simulink model "quindici"  (R2023a)
settings: Solver=VariableStepAuto  StartTime=0.0  StopTime=10*((2*pi)/w)  MaxStep=((2*pi)/w)/1000  RelTol=1e-3
model workspace (MAT data in the model file):
  R1 = 30
  R2 = 15
  R3 = 4
  R4 = 6
  XC = -16
  XL1 = 18
  XL2 = 18
  XM = 9
  a = 2
  w = 6.28318530718
libraries: fl_lib x16, nesl_utility x5
settings Model: Creator=Aguer  LastModifiedBy=Aguer

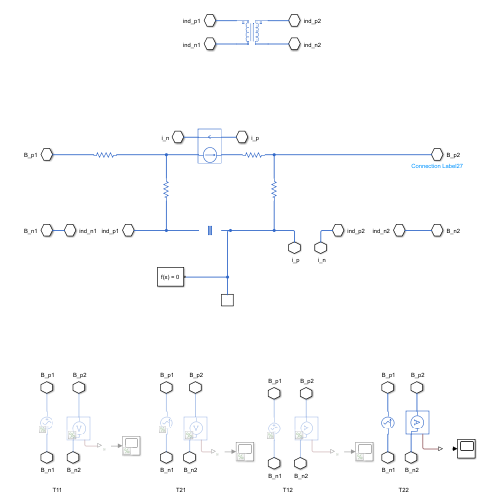
[thumbnail: Simulink's stored preview of the top-level diagram]
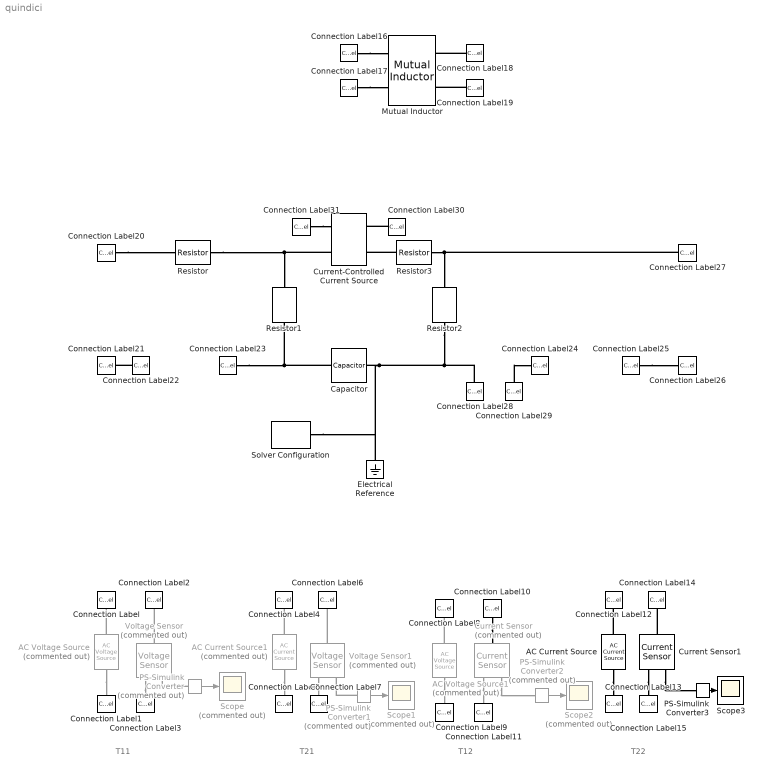
== system quindici ==
  note: T21
  note: T11
  note: T12
  note: T22
  AC Current Source : fl_lib/Electrical/Electrical Sources/AC Current Source  amp=1 A  shift=90 deg  frequency=w/(2*pi) Hz  omega=0 rad/s
      settings: InternalSimscapePortConfiguration="{\"Bottom\":[],\"Left\":[{\"id\":\"p\",\"label\":\"\",\"type\":\"foundation.electrical.electrical\"}],\"Right\":[{\"id\":\"n\",\"label\":\"\",\"type\":\"foundation.electrical.electrical\"}],\"Top\":[]}"
  AC Current Source1 : fl_lib/Electrical/Electrical Sources/AC Current Source  Commented=on  amp=1 A  shift=90 deg  frequency=w/(2*pi) Hz  omega=0 rad/s
      settings: InternalSimscapePortConfiguration="{\"Bottom\":[],\"Left\":[{\"id\":\"p\",\"label\":\"\",\"type\":\"foundation.electrical.electrical\"}],\"Right\":[{\"id\":\"n\",\"label\":\"\",\"type\":\"foundation.electrical.electrical\"}],\"Top\":[]}"
  AC Voltage Source : fl_lib/Electrical/Electrical Sources/AC Voltage Source  Commented=on  amp=1 V  shift=90 deg  frequency=w/(2*pi) Hz  omega=0 rad/s
  AC Voltage Source1 : fl_lib/Electrical/Electrical Sources/AC Voltage Source  Commented=on  amp=1 V  shift=90 deg  frequency=w/(2*pi) Hz  omega=0 rad/s
  Capacitor : fl_lib/Electrical/Electrical Elements/Capacitor  c=-1/(w*XC) F  r=0 Ohm  g=0 1/Ohm  i_specify=off  i_priority=None  i=0 A  i_nominal_specify=off  i_nominal_unit=A  i_nominal_value=1  v_specify=off  v_priority=None  v=0 V  v_nominal_specify=off  v_nominal_unit=V  v_nominal_value=1  vc_specify=off  vc_priority=High  vc=0 V  vc_nominal_specify=off  vc_nominal_unit=V  vc_nominal_value=1
  Connection Label{,4,8,12,20} (5 alike) : ConnectionLabel  Label=B_p1
  Connection Label{1,5,9,13,21} (5 alike) : ConnectionLabel  Label=B_n1
  Connection Label{2,6,10,14,27} (5 alike) : ConnectionLabel  Label=B_p2
  Connection Label{3,7,11,15,26} (5 alike) : ConnectionLabel  Label=B_n2
  Connection Label16 : ConnectionLabel  Label=ind_p1
  Connection Label17 : ConnectionLabel  Label=ind_n1
  Connection Label18 : ConnectionLabel  Label=ind_p2
  Connection Label19 : ConnectionLabel  Label=ind_n2
  Connection Label22 : ConnectionLabel  Label=ind_n1
  Connection Label23 : ConnectionLabel  Label=ind_p1
  Connection Label24 : ConnectionLabel  Label=ind_p2
  Connection Label25 : ConnectionLabel  Label=ind_n2
  Connection Label28 : ConnectionLabel  Label=i_p
  Connection Label29 : ConnectionLabel  Label=i_n
  Connection Label30 : ConnectionLabel  Label=i_p
  Connection Label31 : ConnectionLabel  Label=i_n
  Current Sensor : fl_lib/Electrical/Electrical Sensors/Current Sensor  Commented=on
  Current Sensor1 : fl_lib/Electrical/Electrical Sensors/Current Sensor
  Current-Controlled Current Source : fl_lib/Electrical/Electrical Sources/Current-Controlled Current Source  K=a  i1_specify=off  i1_priority=None  i1=0 A  i1_nominal_specify=off  i1_nominal_unit=A  i1_nominal_value=1  i2_specify=off  i2_priority=None  i2=0 A  i2_nominal_specify=off  i2_nominal_unit=A  i2_nominal_value=1
      settings: InternalSimscapePortConfiguration="{\"Bottom\":[],\"Left\":[{\"id\":\"p1\",\"label\":\"+\",\"type\":\"foundation.electrical.electrical\"},{\"id\":\"head\",\"label\":\"\",\"type\":\"foundation.electrical.electrical\"}],\"Right\":[{\"id\":\"n1\",\"label\":\"-\",\"type\":\"foundation.electrical.electrical\"},{\"id\":\"tail\",\"label\":\"\",\"type\":\"foundation.electrical.electrical\"}],\"Top\":[]}"
  Electrical Reference : fl_lib/Electrical/Electrical Elements/Electrical Reference
  Mutual Inductor : fl_lib/Electrical/Electrical Elements/Mutual Inductor  L1=XL1/w H  L2=XL2/w H  k=XM/XL1  i1_specify=off  i1_priority=High  i1=0 A  i1_nominal_specify=off  i1_nominal_unit=A  i1_nominal_value=1  i2_specify=off  i2_priority=High  i2=0 A  i2_nominal_specify=off  i2_nominal_unit=A  i2_nominal_value=1  v1_specify=off  v1_priority=None  v1=0 V  v1_nominal_specify=off  v1_nominal_unit=V  v1_nominal_value=1  v2_specify=off  v2_priority=None  v2=0 V  v2_nominal_specify=off  v2_nominal_unit=V  v2_nominal_value=1
      settings: InternalSimscapePortConfiguration="{\"Bottom\":[],\"Left\":[{\"id\":\"p1\",\"label\":\"1+\",\"type\":\"foundation.electrical.electrical\"},{\"id\":\"n1\",\"label\":\"1-\",\"type\":\"foundation.electrical.electrical\"}],\"Right\":[{\"id\":\"p2\",\"label\":\"2+\",\"type\":\"foundation.electrical.electrical\"},{\"id\":\"n2\",\"label\":\"2-\",\"type\":\"foundation.electrical.electrical\"}],\"Top\":[]}"
  PS-Simulink Converter : nesl_utility/PS-Simulink Converter  Commented=on  PhysicalDomain=network_engine_domain  SubClassName=ps_output  LeftPortType=input  RightPortType=output  PseudoPeriodic=off  Frequencies=[]  VectorFormat=inherit  Unit=inherit  AffineConversion=off
  PS-Simulink Converter1 : nesl_utility/PS-Simulink Converter  Commented=on  PhysicalDomain=network_engine_domain  SubClassName=ps_output  LeftPortType=input  RightPortType=output  PseudoPeriodic=off  Frequencies=[]  VectorFormat=inherit  Unit=inherit  AffineConversion=off
  PS-Simulink Converter2 : nesl_utility/PS-Simulink Converter  Commented=on  PhysicalDomain=network_engine_domain  SubClassName=ps_output  LeftPortType=input  RightPortType=output  PseudoPeriodic=off  Frequencies=[]  VectorFormat=inherit  Unit=inherit  AffineConversion=off
  PS-Simulink Converter3 : nesl_utility/PS-Simulink Converter  PhysicalDomain=network_engine_domain  SubClassName=ps_output  LeftPortType=input  RightPortType=output  PseudoPeriodic=off  Frequencies=[]  VectorFormat=inherit  Unit=inherit  AffineConversion=off
  Resistor : fl_lib/Electrical/Electrical Elements/Resistor  R=R1 Ohm  i_specify=off  i_priority=None  i=0 A  i_nominal_specify=off  i_nominal_unit=A  i_nominal_value=1  v_specify=off  v_priority=None  v=0 V  v_nominal_specify=off  v_nominal_unit=V  v_nominal_value=1
  Resistor1 : fl_lib/Electrical/Electrical Elements/Resistor  R=R2 Ohm  i_specify=off  i_priority=None  i=0 A  i_nominal_specify=off  i_nominal_unit=A  i_nominal_value=1  v_specify=off  v_priority=None  v=0 V  v_nominal_specify=off  v_nominal_unit=V  v_nominal_value=1
  Resistor2 : fl_lib/Electrical/Electrical Elements/Resistor  R=R4 Ohm  i_specify=off  i_priority=None  i=0 A  i_nominal_specify=off  i_nominal_unit=A  i_nominal_value=1  v_specify=off  v_priority=None  v=0 V  v_nominal_specify=off  v_nominal_unit=V  v_nominal_value=1
  Resistor3 : fl_lib/Electrical/Electrical Elements/Resistor  R=R3 Ohm  i_specify=off  i_priority=None  i=0 A  i_nominal_specify=off  i_nominal_unit=A  i_nominal_value=1  v_specify=off  v_priority=None  v=0 V  v_nominal_specify=off  v_nominal_unit=V  v_nominal_value=1
  Scope : Scope  Commented=on
  Scope1 : Scope  Commented=on
  Scope2 : Scope  Commented=on
  Scope3 : Scope
  Solver Configuration : nesl_utility/Solver Configuration  PhysicalDomain=network_engine_domain  SubClassName=solver  LeftPortType=input  RightPortType=generic  Tones=[]  Harmonics=[]  SimulateNoise=off  Profile=off  UseLocalSampling=off  EnableSwitchedLinearOptims=on  FrequencyDomain=off  UseCCode=off  RelTol=0.001  AbsTol=0.001  MinStep=1e-09  ToWorkspace=off  RevertToSquareIcSolve=off  NumHomotopyIterations=100  PhasorMode=off  PhasorModeNumHarmonics=1  ConsistencySolver=NEWTON_XTOL_AFTER_FTOL  IndexReductionMethod=DerivativeReplacement  DoDC=off  ResidualTolerance=1e-09  ConsistencyTolSource=GLOBAL  ConsistencyAbsTol=0.001  ConsistencyRelTol=0.001  ConsistencyTolFactor=0.001  UseLocalSolver=off  LocalSolverChoice=NE_BACKWARD_EULER_ADVANCER  ResolveIndetEquations=on  FunctionEvalNumThread=1  LocalSolverSampleTime=0.001  DoFixedCost=off  MaxNonlinIter=3  MaxModeIter=2  ComputeImpulses=off  ImpulseIterations=2  LinearAlgebra=auto  LinearAlgebraNumThread=0  EquationFormulation=NE_TIME_EF  DelaysMemoryBudget=1024  AutomaticFiltering=on  FilteringTimeConstant=0.001  PartitionStorageMethod=AS_NEEDED  PartitionMemoryBudget=1024  PartitionMethod=ROBUST
  Voltage Sensor : fl_lib/Electrical/Electrical Sensors/Voltage Sensor  Commented=on
  Voltage Sensor1 : fl_lib/Electrical/Electrical Sensors/Voltage Sensor  Commented=on
  wires:
  PS-Simulink Converter3/1 -> Scope3/1
  PS-Simulink Converter2/1 -> Scope2/1
  PS-Simulink Converter/1 -> Scope/1
  PS-Simulink Converter1/1 -> Scope1/1
  connections:
  AC Voltage Source1/LConn1 -- Connection Label8/LConn1
  Voltage Sensor/LConn1 -- Connection Label2/LConn1
  AC Current Source/RConn1 -- Connection Label13/LConn1
  AC Current Source/LConn1 -- Connection Label12/LConn1
  Connection Label19/LConn1 -- Mutual Inductor/RConn2
  Voltage Sensor/RConn2 -- Connection Label3/LConn1
  Current Sensor1/RConn2 -- Connection Label15/LConn1
  Voltage Sensor1/LConn1 -- Connection Label6/LConn1
  PS-Simulink Converter1/LConn1 -- Voltage Sensor1/RConn1
  Current Sensor1/RConn1 -- PS-Simulink Converter3/LConn1
  AC Voltage Source1/RConn1 -- Connection Label9/LConn1
  Current Sensor/RConn2 -- Connection Label11/LConn1
  AC Current Source1/RConn1 -- Connection Label5/LConn1
  Connection Label16/LConn1 -- Mutual Inductor/LConn1
  Current Sensor/RConn1 -- PS-Simulink Converter2/LConn1
  Connection Label10/LConn1 -- Current Sensor/LConn1
  PS-Simulink Converter/LConn1 -- Voltage Sensor/RConn1
  AC Voltage Source/LConn1 -- Connection Label/LConn1
  Current Sensor1/LConn1 -- Connection Label14/LConn1
  AC Voltage Source/RConn1 -- Connection Label1/LConn1
  Connection Label17/LConn1 -- Mutual Inductor/LConn2
  Voltage Sensor1/RConn2 -- Connection Label7/LConn1
  AC Current Source1/LConn1 -- Connection Label4/LConn1
  Connection Label18/LConn1 -- Mutual Inductor/RConn1
  Resistor/RConn1 -- Resistor1/LConn1 -- Current-Controlled Current Source/RConn2
  Connection Label20/LConn1 -- Resistor/LConn1
  Connection Label22/LConn1 -- Connection Label21/LConn1
  Connection Label23/LConn1 -- Capacitor/LConn1 -- Resistor1/RConn1
  Resistor2/RConn1 -- Connection Label28/LConn1 -- Solver Configuration/RConn1 -- Electrical Reference/LConn1 -- Capacitor/RConn1
  Resistor3/RConn1 -- Connection Label27/LConn1 -- Resistor2/LConn1
  Resistor3/LConn1 -- Current-Controlled Current Source/LConn2
  Connection Label25/LConn1 -- Connection Label26/LConn1
  Connection Label29/LConn1 -- Connection Label24/LConn1
  Connection Label30/LConn1 -- Current-Controlled Current Source/LConn1
  Connection Label31/LConn1 -- Current-Controlled Current Source/RConn1
